simulink model "massDamperSpringModel"  (R2021b)
settings: Solver=ode23s  StartTime=0.0  StopTime=10.0  MaxStep=1e-2  RelTol=1e-3
InitFcn:
  | massDamperSpringInit
values from neighbouring files (symbols this model uses):
  d = modelParams.DAMPER_CONST    [massDamperSpringInit.m]    (also in modelParams.m = 3)
  m = modelParams.MASS    [massDamperSpringInit.m]    (also in modelParams.m = 1)
  s = modelParams.SPRING_CONST    [massDamperSpringInit.m]    (also in modelParams.m = 10)
libraries: stateSpaceMdl x1
settings Model: Creator=feren  LastModifiedBy=Lindenmaier László
settings SolverCC: AlgebraicLoopSolver=TrustRegion
settings DataIOCC: ExternalInput=[modelInput.timeVect, modelInput.inputVect]  LoadExternalInput=on
settings DebuggingCC: SFMachineParentedDataDiag=warning

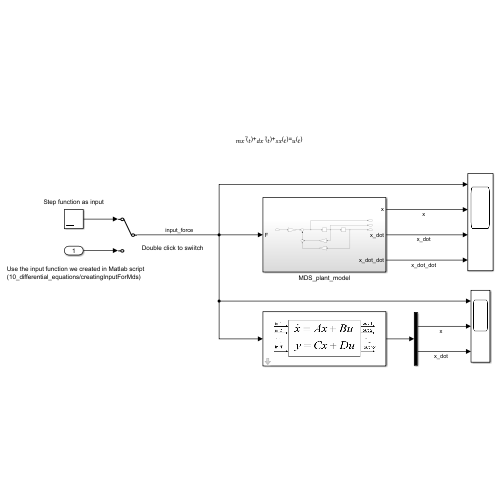
[thumbnail: Simulink's stored preview of the top-level diagram]
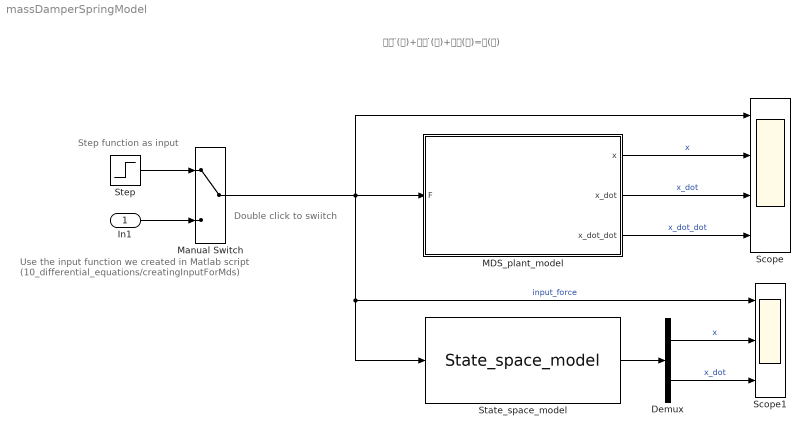
== system massDamperSpringModel ==
  note: Use the input function we created in Matlab script
      | (10_differential_equations/creatingInputForMds)
  note: 𝑚𝑥 ̈(𝑡)+𝑑𝑥 ̇(𝑡)+𝑠𝑥(𝑡)=𝑢(𝑡)
  note: Step function as input
  note: Double click to swiitch
  In1 : Inport
  Demux : Demux  Outputs=2
  MDS_plant_model : Subsystem
  Manual Switch : ManualSwitch
  Scope : Scope  NumInputPorts=4
  Scope1 : Scope  NumInputPorts=3
  State_space_model : stateSpaceMdl/State_space_model  A_in=A_mds  B_in=B_mds
  Step : Step  Time=2  SampleTime=0
  wires:
  Manual Switch/1 -> Scope/1, MDS_plant_model/1(F), Scope1/1, State_space_model/1  "input_force"
  State_space_model/1 -> Demux/1
  Step/1 -> Manual Switch/1
  In1/1 -> Manual Switch/2
  Demux/1 -> Scope1/2  "x"
  Demux/2 -> Scope1/3  "x_dot"
  MDS_plant_model/1(x) -> Scope/2  "x"
  MDS_plant_model/2(x_dot) -> Scope/3  "x_dot"
  MDS_plant_model/3(x_dot_dot) -> Scope/4  "x_dot_dot"

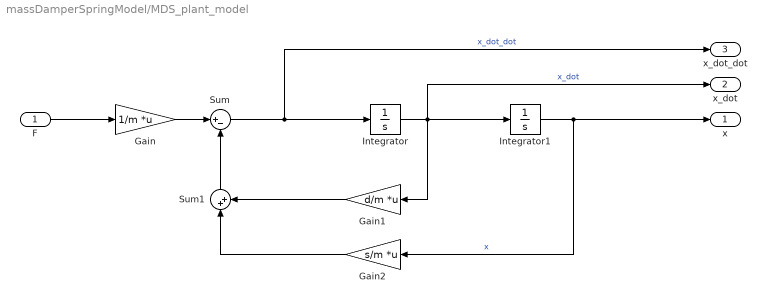
== system massDamperSpringModel/MDS_plant_model ==
  F : Inport
  Gain : Gain  Gain=1/m  Multiplication=Matrix(K*u)
  Gain1 : Gain  Gain=d/m  Multiplication=Matrix(K*u)
  Gain2 : Gain  Gain=s/m  Multiplication=Matrix(K*u)
  Integrator : Integrator
  Integrator1 : Integrator
  Sum : Sum  Inputs=|+-
  Sum1 : Sum  Inputs=|++
  x : Outport
  x_dot : Outport  Port=2
  x_dot_dot : Outport  Port=3
  wires:
  Gain2/1 -> Sum1/1
  Gain/1 -> Sum/1
  Integrator1/1 -> x/1, Gain2/1  "x"
  Integrator/1 -> x_dot/1, Gain1/1, Integrator1/1  "x_dot"
  Gain1/1 -> Sum1/2
  Sum/1 -> Integrator/1, x_dot_dot/1  "x_dot_dot"
  Sum1/1 -> Sum/2
  F/1 -> Gain/1
